simulink model "GPESTN1"  (Simulink 6.1)
settings: Solver=ode45  StartTime=0.0  StopTime=1000.0  MaxStep=0.02  MinStep=0.005  RelTol=1e-3
values from neighbouring files (symbols this model uses):
  A_gpe = 2    [data_GPE.m]    (also in data_GPI.m)
  A_stn = 5    [data_GPI.m]    (also in data_STN.m)
  B_gpe = .08    (= 0.08)    [data_GPE.m]    (also in data_GPI.m)
  B_stn = 1    [data_GPI.m]    (also in data_STN.m)
  c_gpe = 1    [data_GPE.m]
  c_stn = 1    [data_STN.m]
  cag0 = i_v_16(177:192)    [launch_sysGPESTN1.m]    (also in launch_sysGPESTN1_GPEDBS.m)
  cas0 = i_v_16(65:80)    [launch_sysGPESTN1.m]    (also in launch_sysGPESTN1_GPEDBS.m)
  egpegpe = -80    [data_synapses.m]
  egpestn = -100    [data_synapses.m]
  ek_gpe = -80.0    (= -80)    [data_GPE.m]
  ek_stn = -80.0    (= -80)    [data_STN.m]
  el_gpe = -55.0    (= -55)    [data_GPE.m]
  el_stn = -60.0    (= -60)    [data_STN.m]
  epsil_gpe = 1*10^-4    (= 0.0001)    [data_GPE.m]
  epsil_stn = 3.75*10^-5    (= 3.75e-05)    [data_STN.m]
  estngpe = 0    [data_synapses.m]
  gahp_gpe = 30.0    (= 30)    [data_GPE.m]
  gahp_stn = 9.0    (= 9)    [data_STN.m]
  gca_gpe = 0.1    [data_GPE.m]
  gca_stn = 0.5    [data_STN.m]
  ggpegpe = .3    (= 0.3)    [data_synapses.m]    (also in launch_sysGPESTN1.m; launch_sysGPESTN1_GPEDBS.m = 0)
  ggpestn = .90    (= 0.9)    [data_synapses.m]
  gk_gpe = 30.0    (= 30)    [data_GPE.m]
  gk_stn = 45.0    (= 45)    [data_STN.m]
  gl_gpe = .1    (= 0.1)    [data_GPE.m]
  gl_stn = 2.25    [data_STN.m]
  gna_gpe = 120    [data_GPE.m]
  gna_stn = 37.5    [data_STN.m]
  gstngpe = .3    (= 0.3)    [data_synapses.m]
  gt_gpe = .5    (= 0.5)    [data_GPE.m]
  gt_stn = 0.5    [data_STN.m]
  hg0 = i_v_16(129:144)    [launch_sysGPESTN1.m]    (also in launch_sysGPESTN1_GPEDBS.m)
  hs0 = i_v_16(17:32)    [launch_sysGPESTN1.m]    (also in launch_sysGPESTN1_GPEDBS.m)
  k1_gpe = 30.0    (= 30)    [data_GPE.m]
  k1_stn = 15.0    (= 15)    [data_STN.m]
  kca_gpe = 15    [data_GPE.m]
  kca_stn = 22.5    [data_STN.m]
  ng0 = i_v_16(145:160)    [launch_sysGPESTN1.m]    (also in launch_sysGPESTN1_GPEDBS.m)
  ns0 = i_v_16(33:48)    [launch_sysGPESTN1.m]    (also in launch_sysGPESTN1_GPEDBS.m)
  phih_gpe = 0.05    [data_GPE.m]
  phih_stn = 0.75    [data_STN.m]
  phin_gpe = 0.1    [data_GPE.m]
  phin_stn = 0.75    [data_STN.m]
  phir_gpe = 1    [data_GPE.m]
  phir_stn = 0.5    [data_STN.m]
  rg0 = i_v_16(161:176)    [launch_sysGPESTN1.m]    (also in launch_sysGPESTN1_GPEDBS.m)
  rs0 = i_v_16(49:64)    [launch_sysGPESTN1.m]    (also in launch_sysGPESTN1_GPEDBS.m)
  sg0 = i_v_16(193:208)    [launch_sysGPESTN1.m]    (also in launch_sysGPESTN1_GPEDBS.m)
  sigmaa_gpe = 2    [data_GPE.m]
  sigmaa_stn = 7.8    [data_STN.m]
  sigmab_stn = -0.07    [data_STN.m]
  sigmagh_gpe = 2.0    (= 2)    [data_GPE.m]
  sigmagh_stn = 8.0    (= 8)    [data_STN.m]
  sigmah_gpe = -12    [data_GPE.m]
  sigmah_stn = -3.1    [data_STN.m]
  sigmam_gpe = 10.0    (= 10)    [data_GPE.m]
  sigmam_stn = 15.0    (= 15)    [data_STN.m]
  sigman_gpe = 14.0    (= 14)    [data_GPE.m]
  sigman_stn = 8.0    (= 8)    [data_STN.m]
  sigmar_gpe = -2.0    (= -2)    [data_GPE.m]
  sigmar_stn = -2.0    (= -2)    [data_STN.m]
  sigmas_gpe = 2    [data_GPE.m]
  sigmas_stn = 8.0    (= 8)    [data_STN.m]
  sigmatauh_gpe = -12    [data_GPE.m]
  sigmatauh_stn = -3.0    (= -3)    [data_STN.m]
  sigmataun_gpe = -12.0    (= -12)    [data_GPE.m]
  sigmataun_stn = -26.0    (= -26)    [data_STN.m]
  sigmataur_stn = -2.2    [data_STN.m]
  ss0 = i_v_16(81:96)    [launch_sysGPESTN1.m]    (also in launch_sysGPESTN1_GPEDBS.m)
  syn_stngpe_gain = .2    (= 0.2)    [data_STN.m]
  tauh0_gpe = .05    (= 0.05)    [data_GPE.m]
  tauh0_stn = 1.0    (= 1)    [data_STN.m]
  tauh1_gpe = .27    (= 0.27)    [data_GPE.m]
  tauh1_stn = 500.0    (= 500)    [data_STN.m]
  taun0_gpe = .05    (= 0.05)    [data_GPE.m]
  taun0_stn = 1.0    (= 1)    [data_STN.m]
  taun1_gpe = .27    (= 0.27)    [data_GPE.m]
  taun1_stn = 100.0    (= 100)    [data_STN.m]
  taur0_stn = 7.1    [data_STN.m]
  taur1_stn = 17.5    [data_STN.m]
  taur_gpe = 30.0    (= 30)    [data_GPE.m]
  theta_gpe = 20    [data_GPE.m]    (also in data_GPI.m)
  theta_stn = 30    [data_GPI.m]    (also in data_STN.m)
  thetaa_gpe = -57.0    (= -57)    [data_GPE.m]
  thetaa_stn = -63.0    (= -63)    [data_STN.m]
  thetab_stn = 0.25    [data_STN.m]
  thetagh_gpe = -57.0    (= -57)    [data_GPE.m]
  thetagh_stn = -39.0    (= -39)    [data_STN.m]
  thetah_gpe = -58.0    (= -58)    [data_GPE.m]
  thetah_stn = -39.0    (= -39)    [data_STN.m]
  thetam_gpe = -37.0    (= -37)    [data_GPE.m]
  thetam_stn = -30.0    (= -30)    [data_STN.m]
  thetan_gpe = -50.0    (= -50)    [data_GPE.m]
  thetan_stn = -32.0    (= -32)    [data_STN.m]
  thetar_gpe = -70.0    (= -70)    [data_GPE.m]
  thetar_stn = -67.0    (= -67)    [data_STN.m]
  thetas_gpe = -35.0    (= -35)    [data_GPE.m]
  thetas_stn = -39.0    (= -39)    [data_STN.m]
  thetatauh_gpe = -40.0    (= -40)    [data_GPE.m]
  thetatauh_stn = -57.0    (= -57)    [data_STN.m]
  thetataun_gpe = -40.0    (= -40)    [data_GPE.m]
  thetataun_stn = -80.0    (= -80)    [data_STN.m]
  thetataur_stn = 68.0    (= 68)    [data_STN.m]
  vg0 = i_v_16(113:128)    [launch_sysGPESTN1.m]    (also in launch_sysGPESTN1_GPEDBS.m)
  vs0 = i_v_16(1:16)    [launch_sysGPESTN1.m]    (also in launch_sysGPESTN1_GPEDBS.m)
undefined symbols (not defined in the file or in its folder): cag01, cas01, hg01, hs01, ng01, ns01, rg01, rs01, sg01, ss01, vg01, vs01
(part 2 of 9)

== system GPESTN1/igpegpe4 ==
  In1 : Inport  Port=1  LatchInput=off
  In2 : Inport  Port=2  LatchInput=off
  In3 : Inport  Port=3  LatchInput=off
  Fcn : Fcn  Expr=ggpegpe*(u-egpegpe)
  Product : Product  SaturateOnIntegerOverflow=on  InputSameDT=on
  Sum : Sum  SaturateOnIntegerOverflow=on  InputSameDT=on
  Out1 : Outport
  wires:
  Sum/1 -> Product/1
  Fcn/1 -> Product/2
  In1/1 -> Sum/1
  In2/1 -> Sum/2
  Product/1 -> Out1/1
  In3/1 -> Fcn/1

== system GPESTN1/igpegpe5 ==
  In1 : Inport  Port=1  LatchInput=off
  In2 : Inport  Port=2  LatchInput=off
  In3 : Inport  Port=3  LatchInput=off
  Fcn : Fcn  Expr=ggpegpe*(u-egpegpe)
  Product : Product  SaturateOnIntegerOverflow=on  InputSameDT=on
  Sum : Sum  SaturateOnIntegerOverflow=on  InputSameDT=on
  Out1 : Outport
  wires:
  Sum/1 -> Product/1
  Fcn/1 -> Product/2
  In1/1 -> Sum/1
  In2/1 -> Sum/2
  Product/1 -> Out1/1
  In3/1 -> Fcn/1

== system GPESTN1/igpegpe6 ==
  In1 : Inport  Port=1  LatchInput=off
  In2 : Inport  Port=2  LatchInput=off
  In3 : Inport  Port=3  LatchInput=off
  Fcn : Fcn  Expr=ggpegpe*(u-egpegpe)
  Product : Product  SaturateOnIntegerOverflow=on  InputSameDT=on
  Sum : Sum  SaturateOnIntegerOverflow=on  InputSameDT=on
  Out1 : Outport
  wires:
  Sum/1 -> Product/1
  Fcn/1 -> Product/2
  In1/1 -> Sum/1
  In2/1 -> Sum/2
  Product/1 -> Out1/1
  In3/1 -> Fcn/1

== system GPESTN1/igpegpe7 ==
  In1 : Inport  Port=1  LatchInput=off
  In2 : Inport  Port=2  LatchInput=off
  In3 : Inport  Port=3  LatchInput=off
  Fcn : Fcn  Expr=ggpegpe*(u-egpegpe)
  Product : Product  SaturateOnIntegerOverflow=on  InputSameDT=on
  Sum : Sum  SaturateOnIntegerOverflow=on  InputSameDT=on
  Out1 : Outport
  wires:
  Sum/1 -> Product/1
  Fcn/1 -> Product/2
  In1/1 -> Sum/1
  In2/1 -> Sum/2
  Product/1 -> Out1/1
  In3/1 -> Fcn/1

== system GPESTN1/igpegpe8 ==
  In1 : Inport  Port=1  LatchInput=off
  In2 : Inport  Port=2  LatchInput=off
  In3 : Inport  Port=3  LatchInput=off
  Fcn : Fcn  Expr=ggpegpe*(u-egpegpe)
  Product : Product  SaturateOnIntegerOverflow=on  InputSameDT=on
  Sum : Sum  SaturateOnIntegerOverflow=on  InputSameDT=on
  Out1 : Outport
  wires:
  Sum/1 -> Product/1
  Fcn/1 -> Product/2
  In1/1 -> Sum/1
  In2/1 -> Sum/2
  Product/1 -> Out1/1
  In3/1 -> Fcn/1

== system GPESTN1/igpegpe9 ==
  In1 : Inport  Port=1  LatchInput=off
  In2 : Inport  Port=2  LatchInput=off
  In3 : Inport  Port=3  LatchInput=off
  Fcn : Fcn  Expr=ggpegpe*(u-egpegpe)
  Product : Product  SaturateOnIntegerOverflow=on  InputSameDT=on
  Sum : Sum  SaturateOnIntegerOverflow=on  InputSameDT=on
  Out1 : Outport
  wires:
  Sum/1 -> Product/1
  Fcn/1 -> Product/2
  In1/1 -> Sum/1
  In2/1 -> Sum/2
  Product/1 -> Out1/1
  In3/1 -> Fcn/1

== system GPESTN1/igpestn ==
  In1 : Inport  Port=1  LatchInput=off
  In2 : Inport  Port=2  LatchInput=off
  In3 : Inport  Port=3  LatchInput=off
  Fcn : Fcn  Expr=ggpestn*(u-egpestn)
  Product : Product  SaturateOnIntegerOverflow=on  InputSameDT=on
  Sum : Sum  SaturateOnIntegerOverflow=on  InputSameDT=on
  Out1 : Outport
  wires:
  Sum/1 -> Product/1
  Fcn/1 -> Product/2
  In1/1 -> Sum/1
  In2/1 -> Sum/2
  Product/1 -> Out1/1
  In3/1 -> Fcn/1

== system GPESTN1/igpestn1 ==
  In1 : Inport  Port=1  LatchInput=off
  In2 : Inport  Port=2  LatchInput=off
  In3 : Inport  Port=3  LatchInput=off
  Fcn : Fcn  Expr=ggpestn*(u-egpestn)
  Product : Product  SaturateOnIntegerOverflow=on  InputSameDT=on
  Sum : Sum  SaturateOnIntegerOverflow=on  InputSameDT=on
  Out1 : Outport
  wires:
  Sum/1 -> Product/1
  Fcn/1 -> Product/2
  In1/1 -> Sum/1
  In2/1 -> Sum/2
  Product/1 -> Out1/1
  In3/1 -> Fcn/1

== system GPESTN1/igpestn10 ==
  In1 : Inport  Port=1  LatchInput=off
  In2 : Inport  Port=2  LatchInput=off
  In3 : Inport  Port=3  LatchInput=off
  Fcn : Fcn  Expr=ggpestn*(u-egpestn)
  Product : Product  SaturateOnIntegerOverflow=on  InputSameDT=on
  Sum : Sum  SaturateOnIntegerOverflow=on  InputSameDT=on
  Out1 : Outport
  wires:
  Sum/1 -> Product/1
  Fcn/1 -> Product/2
  In1/1 -> Sum/1
  In2/1 -> Sum/2
  Product/1 -> Out1/1
  In3/1 -> Fcn/1

== system GPESTN1/igpestn11 ==
  In1 : Inport  Port=1  LatchInput=off
  In2 : Inport  Port=2  LatchInput=off
  In3 : Inport  Port=3  LatchInput=off
  Fcn : Fcn  Expr=ggpestn*(u-egpestn)
  Product : Product  SaturateOnIntegerOverflow=on  InputSameDT=on
  Sum : Sum  SaturateOnIntegerOverflow=on  InputSameDT=on
  Out1 : Outport
  wires:
  Sum/1 -> Product/1
  Fcn/1 -> Product/2
  In1/1 -> Sum/1
  In2/1 -> Sum/2
  Product/1 -> Out1/1
  In3/1 -> Fcn/1

== system GPESTN1/igpestn12 ==
  In1 : Inport  Port=1  LatchInput=off
  In2 : Inport  Port=2  LatchInput=off
  In3 : Inport  Port=3  LatchInput=off
  Fcn : Fcn  Expr=ggpestn*(u-egpestn)
  Product : Product  SaturateOnIntegerOverflow=on  InputSameDT=on
  Sum : Sum  SaturateOnIntegerOverflow=on  InputSameDT=on
  Out1 : Outport
  wires:
  Sum/1 -> Product/1
  Fcn/1 -> Product/2
  In1/1 -> Sum/1
  In2/1 -> Sum/2
  Product/1 -> Out1/1
  In3/1 -> Fcn/1

== system GPESTN1/igpestn13 ==
  In1 : Inport  Port=1  LatchInput=off
  In2 : Inport  Port=2  LatchInput=off
  In3 : Inport  Port=3  LatchInput=off
  Fcn : Fcn  Expr=ggpestn*(u-egpestn)
  Product : Product  SaturateOnIntegerOverflow=on  InputSameDT=on
  Sum : Sum  SaturateOnIntegerOverflow=on  InputSameDT=on
  Out1 : Outport
  wires:
  Sum/1 -> Product/1
  Fcn/1 -> Product/2
  In1/1 -> Sum/1
  In2/1 -> Sum/2
  Product/1 -> Out1/1
  In3/1 -> Fcn/1

== system GPESTN1/igpestn14 ==
  In1 : Inport  Port=1  LatchInput=off
  In2 : Inport  Port=2  LatchInput=off
  In3 : Inport  Port=3  LatchInput=off
  Fcn : Fcn  Expr=ggpestn*(u-egpestn)
  Product : Product  SaturateOnIntegerOverflow=on  InputSameDT=on
  Sum : Sum  SaturateOnIntegerOverflow=on  InputSameDT=on
  Out1 : Outport
  wires:
  Sum/1 -> Product/1
  Fcn/1 -> Product/2
  In1/1 -> Sum/1
  In2/1 -> Sum/2
  Product/1 -> Out1/1
  In3/1 -> Fcn/1

== system GPESTN1/igpestn15 ==
  In1 : Inport  Port=1  LatchInput=off
  In2 : Inport  Port=2  LatchInput=off
  In3 : Inport  Port=3  LatchInput=off
  Fcn : Fcn  Expr=ggpestn*(u-egpestn)
  Product : Product  SaturateOnIntegerOverflow=on  InputSameDT=on
  Sum : Sum  SaturateOnIntegerOverflow=on  InputSameDT=on
  Out1 : Outport
  wires:
  Sum/1 -> Product/1
  Fcn/1 -> Product/2
  In1/1 -> Sum/1
  In2/1 -> Sum/2
  Product/1 -> Out1/1
  In3/1 -> Fcn/1

== system GPESTN1/igpestn2 ==
  In1 : Inport  Port=1  LatchInput=off
  In2 : Inport  Port=2  LatchInput=off
  In3 : Inport  Port=3  LatchInput=off
  Fcn : Fcn  Expr=ggpestn*(u-egpestn)
  Product : Product  SaturateOnIntegerOverflow=on  InputSameDT=on
  Sum : Sum  SaturateOnIntegerOverflow=on  InputSameDT=on
  Out1 : Outport
  wires:
  Sum/1 -> Product/1
  Fcn/1 -> Product/2
  In1/1 -> Sum/1
  In2/1 -> Sum/2
  Product/1 -> Out1/1
  In3/1 -> Fcn/1

== system GPESTN1/igpestn3 ==
  In1 : Inport  Port=1  LatchInput=off
  In2 : Inport  Port=2  LatchInput=off
  In3 : Inport  Port=3  LatchInput=off
  Fcn : Fcn  Expr=ggpestn*(u-egpestn)
  Product : Product  SaturateOnIntegerOverflow=on  InputSameDT=on
  Sum : Sum  SaturateOnIntegerOverflow=on  InputSameDT=on
  Out1 : Outport
  wires:
  Sum/1 -> Product/1
  Fcn/1 -> Product/2
  In1/1 -> Sum/1
  In2/1 -> Sum/2
  Product/1 -> Out1/1
  In3/1 -> Fcn/1

== system GPESTN1/igpestn4 ==
  In1 : Inport  Port=1  LatchInput=off
  In2 : Inport  Port=2  LatchInput=off
  In3 : Inport  Port=3  LatchInput=off
  Fcn : Fcn  Expr=ggpestn*(u-egpestn)
  Product : Product  SaturateOnIntegerOverflow=on  InputSameDT=on
  Sum : Sum  SaturateOnIntegerOverflow=on  InputSameDT=on
  Out1 : Outport
  wires:
  Sum/1 -> Product/1
  Fcn/1 -> Product/2
  In1/1 -> Sum/1
  In2/1 -> Sum/2
  Product/1 -> Out1/1
  In3/1 -> Fcn/1

== system GPESTN1/igpestn5 ==
  In1 : Inport  Port=1  LatchInput=off
  In2 : Inport  Port=2  LatchInput=off
  In3 : Inport  Port=3  LatchInput=off
  Fcn : Fcn  Expr=ggpestn*(u-egpestn)
  Product : Product  SaturateOnIntegerOverflow=on  InputSameDT=on
  Sum : Sum  SaturateOnIntegerOverflow=on  InputSameDT=on
  Out1 : Outport
  wires:
  Sum/1 -> Product/1
  Fcn/1 -> Product/2
  In1/1 -> Sum/1
  In2/1 -> Sum/2
  Product/1 -> Out1/1
  In3/1 -> Fcn/1

== system GPESTN1/igpestn6 ==
  In1 : Inport  Port=1  LatchInput=off
  In2 : Inport  Port=2  LatchInput=off
  In3 : Inport  Port=3  LatchInput=off
  Fcn : Fcn  Expr=ggpestn*(u-egpestn)
  Product : Product  SaturateOnIntegerOverflow=on  InputSameDT=on
  Sum : Sum  SaturateOnIntegerOverflow=on  InputSameDT=on
  Out1 : Outport
  wires:
  Sum/1 -> Product/1
  Fcn/1 -> Product/2
  In1/1 -> Sum/1
  In2/1 -> Sum/2
  Product/1 -> Out1/1
  In3/1 -> Fcn/1

== system GPESTN1/igpestn7 ==
  In1 : Inport  Port=1  LatchInput=off
  In2 : Inport  Port=2  LatchInput=off
  In3 : Inport  Port=3  LatchInput=off
  Fcn : Fcn  Expr=ggpestn*(u-egpestn)
  Product : Product  SaturateOnIntegerOverflow=on  InputSameDT=on
  Sum : Sum  SaturateOnIntegerOverflow=on  InputSameDT=on
  Out1 : Outport
  wires:
  Sum/1 -> Product/1
  Fcn/1 -> Product/2
  In1/1 -> Sum/1
  In2/1 -> Sum/2
  Product/1 -> Out1/1
  In3/1 -> Fcn/1

== system GPESTN1/igpestn8 ==
  In1 : Inport  Port=1  LatchInput=off
  In2 : Inport  Port=2  LatchInput=off
  In3 : Inport  Port=3  LatchInput=off
  Fcn : Fcn  Expr=ggpestn*(u-egpestn)
  Product : Product  SaturateOnIntegerOverflow=on  InputSameDT=on
  Sum : Sum  SaturateOnIntegerOverflow=on  InputSameDT=on
  Out1 : Outport
  wires:
  Sum/1 -> Product/1
  Fcn/1 -> Product/2
  In1/1 -> Sum/1
  In2/1 -> Sum/2
  Product/1 -> Out1/1
  In3/1 -> Fcn/1

== system GPESTN1/igpestn9 ==
  In1 : Inport  Port=1  LatchInput=off
  In2 : Inport  Port=2  LatchInput=off
  In3 : Inport  Port=3  LatchInput=off
  Fcn : Fcn  Expr=ggpestn*(u-egpestn)
  Product : Product  SaturateOnIntegerOverflow=on  InputSameDT=on
  Sum : Sum  SaturateOnIntegerOverflow=on  InputSameDT=on
  Out1 : Outport
  wires:
  Sum/1 -> Product/1
  Fcn/1 -> Product/2
  In1/1 -> Sum/1
  In2/1 -> Sum/2
  Product/1 -> Out1/1
  In3/1 -> Fcn/1

== system GPESTN1/istngpe1 ==
  In1 : Inport  Port=1  LatchInput=off
  In2 : Inport  Port=2  LatchInput=off
  In3 : Inport  Port=3  LatchInput=off
  In4 : Inport  Port=4  LatchInput=off
  Fcn : Fcn  Expr=gstngpe*(u-estngpe)
  Gain : Gain  Gain=syn_stngpe_gain
  Product : Product  SaturateOnIntegerOverflow=on  InputSameDT=on
  Sum : Sum  Inputs=+++  SaturateOnIntegerOverflow=on
  Out1 : Outport
  wires:
  Product/1 -> Out1/1
  In1/1 -> Fcn/1
  Fcn/1 -> Product/1
  In2/1 -> Sum/1
  Sum/1 -> Product/2
  In4/1 -> Sum/3
  Gain/1 -> Sum/2
  In3/1 -> Gain/1

== system GPESTN1/istngpe10 ==
  In1 : Inport  Port=1  LatchInput=off
  In2 : Inport  Port=2  LatchInput=off
  In3 : Inport  Port=3  LatchInput=off
  In4 : Inport  Port=4  LatchInput=off
  Fcn : Fcn  Expr=gstngpe*(u-estngpe)
  Gain : Gain  Gain=syn_stngpe_gain
  Product : Product  SaturateOnIntegerOverflow=on  InputSameDT=on
  Sum : Sum  Inputs=+++  SaturateOnIntegerOverflow=on
  Out1 : Outport
  wires:
  Product/1 -> Out1/1
  In1/1 -> Fcn/1
  Fcn/1 -> Product/1
  In2/1 -> Sum/1
  Sum/1 -> Product/2
  In4/1 -> Sum/3
  Gain/1 -> Sum/2
  In3/1 -> Gain/1

== system GPESTN1/istngpe11 ==
  In1 : Inport  Port=1  LatchInput=off
  In2 : Inport  Port=2  LatchInput=off
  In3 : Inport  Port=3  LatchInput=off
  In4 : Inport  Port=4  LatchInput=off
  Fcn : Fcn  Expr=gstngpe*(u-estngpe)
  Gain : Gain  Gain=syn_stngpe_gain
  Product : Product  SaturateOnIntegerOverflow=on  InputSameDT=on
  Sum : Sum  Inputs=+++  SaturateOnIntegerOverflow=on
  Out1 : Outport
  wires:
  Product/1 -> Out1/1
  In1/1 -> Fcn/1
  Fcn/1 -> Product/1
  In2/1 -> Sum/1
  Sum/1 -> Product/2
  In4/1 -> Sum/3
  Gain/1 -> Sum/2
  In3/1 -> Gain/1

== system GPESTN1/istngpe12 ==
  In1 : Inport  Port=1  LatchInput=off
  In2 : Inport  Port=2  LatchInput=off
  In3 : Inport  Port=3  LatchInput=off
  In4 : Inport  Port=4  LatchInput=off
  Fcn : Fcn  Expr=gstngpe*(u-estngpe)
  Gain : Gain  Gain=syn_stngpe_gain
  Product : Product  SaturateOnIntegerOverflow=on  InputSameDT=on
  Sum : Sum  Inputs=+++  SaturateOnIntegerOverflow=on
  Out1 : Outport
  wires:
  Product/1 -> Out1/1
  In1/1 -> Fcn/1
  Fcn/1 -> Product/1
  In2/1 -> Sum/1
  Sum/1 -> Product/2
  In4/1 -> Sum/3
  Gain/1 -> Sum/2
  In3/1 -> Gain/1

== system GPESTN1/istngpe13 ==
  In1 : Inport  Port=1  LatchInput=off
  In2 : Inport  Port=2  LatchInput=off
  In3 : Inport  Port=3  LatchInput=off
  In4 : Inport  Port=4  LatchInput=off
  Fcn : Fcn  Expr=gstngpe*(u-estngpe)
  Gain : Gain  Gain=syn_stngpe_gain
  Product : Product  SaturateOnIntegerOverflow=on  InputSameDT=on
  Sum : Sum  Inputs=+++  SaturateOnIntegerOverflow=on
  Out1 : Outport
  wires:
  Product/1 -> Out1/1
  In1/1 -> Fcn/1
  Fcn/1 -> Product/1
  In2/1 -> Sum/1
  Sum/1 -> Product/2
  In4/1 -> Sum/3
  Gain/1 -> Sum/2
  In3/1 -> Gain/1

== system GPESTN1/istngpe14 ==
  In1 : Inport  Port=1  LatchInput=off
  In2 : Inport  Port=2  LatchInput=off
  In3 : Inport  Port=3  LatchInput=off
  In4 : Inport  Port=4  LatchInput=off
  Fcn : Fcn  Expr=gstngpe*(u-estngpe)
  Gain : Gain  Gain=syn_stngpe_gain
  Product : Product  SaturateOnIntegerOverflow=on  InputSameDT=on
  Sum : Sum  Inputs=+++  SaturateOnIntegerOverflow=on
  Out1 : Outport
  wires:
  Product/1 -> Out1/1
  In1/1 -> Fcn/1
  Fcn/1 -> Product/1
  In2/1 -> Sum/1
  Sum/1 -> Product/2
  In4/1 -> Sum/3
  Gain/1 -> Sum/2
  In3/1 -> Gain/1

== system GPESTN1/istngpe15 ==
  In1 : Inport  Port=1  LatchInput=off
  In2 : Inport  Port=2  LatchInput=off
  In3 : Inport  Port=3  LatchInput=off
  In4 : Inport  Port=4  LatchInput=off
  Fcn : Fcn  Expr=gstngpe*(u-estngpe)
  Gain : Gain  Gain=syn_stngpe_gain
  Product : Product  SaturateOnIntegerOverflow=on  InputSameDT=on
  Sum : Sum  Inputs=+++  SaturateOnIntegerOverflow=on
  Out1 : Outport
  wires:
  Product/1 -> Out1/1
  In1/1 -> Fcn/1
  Fcn/1 -> Product/1
  In2/1 -> Sum/1
  Sum/1 -> Product/2
  In4/1 -> Sum/3
  Gain/1 -> Sum/2
  In3/1 -> Gain/1

== system GPESTN1/istngpe16 ==
  In1 : Inport  Port=1  LatchInput=off
  In2 : Inport  Port=2  LatchInput=off
  In3 : Inport  Port=3  LatchInput=off
  In4 : Inport  Port=4  LatchInput=off
  Fcn : Fcn  Expr=gstngpe*(u-estngpe)
  Gain : Gain  Gain=syn_stngpe_gain
  Product : Product  SaturateOnIntegerOverflow=on  InputSameDT=on
  Sum : Sum  Inputs=+++  SaturateOnIntegerOverflow=on
  Out1 : Outport
  wires:
  Product/1 -> Out1/1
  In1/1 -> Fcn/1
  Fcn/1 -> Product/1
  In2/1 -> Sum/1
  Sum/1 -> Product/2
  In4/1 -> Sum/3
  Gain/1 -> Sum/2
  In3/1 -> Gain/1

== system GPESTN1/istngpe2 ==
  In1 : Inport  Port=1  LatchInput=off
  In2 : Inport  Port=2  LatchInput=off
  In3 : Inport  Port=3  LatchInput=off
  In4 : Inport  Port=4  LatchInput=off
  Fcn : Fcn  Expr=gstngpe*(u-estngpe)
  Gain : Gain  Gain=syn_stngpe_gain
  Product : Product  SaturateOnIntegerOverflow=on  InputSameDT=on
  Sum : Sum  Inputs=+++  SaturateOnIntegerOverflow=on
  Out1 : Outport
  wires:
  Product/1 -> Out1/1
  In1/1 -> Fcn/1
  Fcn/1 -> Product/1
  In2/1 -> Sum/1
  Sum/1 -> Product/2
  In4/1 -> Sum/3
  Gain/1 -> Sum/2
  In3/1 -> Gain/1

== system GPESTN1/istngpe3 ==
  In1 : Inport  Port=1  LatchInput=off
  In2 : Inport  Port=2  LatchInput=off
  In3 : Inport  Port=3  LatchInput=off
  In4 : Inport  Port=4  LatchInput=off
  Fcn : Fcn  Expr=gstngpe*(u-estngpe)
  Gain : Gain  Gain=syn_stngpe_gain
  Product : Product  SaturateOnIntegerOverflow=on  InputSameDT=on
  Sum : Sum  Inputs=+++  SaturateOnIntegerOverflow=on
  Out1 : Outport
  wires:
  Product/1 -> Out1/1
  In1/1 -> Fcn/1
  Fcn/1 -> Product/1
  In2/1 -> Sum/1
  Sum/1 -> Product/2
  In4/1 -> Sum/3
  Gain/1 -> Sum/2
  In3/1 -> Gain/1

== system GPESTN1/istngpe4 ==
  In1 : Inport  Port=1  LatchInput=off
  In2 : Inport  Port=2  LatchInput=off
  In3 : Inport  Port=3  LatchInput=off
  In4 : Inport  Port=4  LatchInput=off
  Fcn : Fcn  Expr=gstngpe*(u-estngpe)
  Gain : Gain  Gain=syn_stngpe_gain
  Product : Product  SaturateOnIntegerOverflow=on  InputSameDT=on
  Sum : Sum  Inputs=+++  SaturateOnIntegerOverflow=on
  Out1 : Outport
  wires:
  Product/1 -> Out1/1
  In1/1 -> Fcn/1
  Fcn/1 -> Product/1
  In2/1 -> Sum/1
  Sum/1 -> Product/2
  In4/1 -> Sum/3
  Gain/1 -> Sum/2
  In3/1 -> Gain/1

== system GPESTN1/istngpe5 ==
  In1 : Inport  Port=1  LatchInput=off
  In2 : Inport  Port=2  LatchInput=off
  In3 : Inport  Port=3  LatchInput=off
  In4 : Inport  Port=4  LatchInput=off
  Fcn : Fcn  Expr=gstngpe*(u-estngpe)
  Gain : Gain  Gain=syn_stngpe_gain
  Product : Product  SaturateOnIntegerOverflow=on  InputSameDT=on
  Sum : Sum  Inputs=+++  SaturateOnIntegerOverflow=on
  Out1 : Outport
  wires:
  Product/1 -> Out1/1
  In1/1 -> Fcn/1
  Fcn/1 -> Product/1
  In2/1 -> Sum/1
  Sum/1 -> Product/2
  In4/1 -> Sum/3
  Gain/1 -> Sum/2
  In3/1 -> Gain/1

== system GPESTN1/istngpe6 ==
  In1 : Inport  Port=1  LatchInput=off
  In2 : Inport  Port=2  LatchInput=off
  In3 : Inport  Port=3  LatchInput=off
  In4 : Inport  Port=4  LatchInput=off
  Fcn : Fcn  Expr=gstngpe*(u-estngpe)
  Gain : Gain  Gain=syn_stngpe_gain
  Product : Product  SaturateOnIntegerOverflow=on  InputSameDT=on
  Sum : Sum  Inputs=+++  SaturateOnIntegerOverflow=on
  Out1 : Outport
  wires:
  Product/1 -> Out1/1
  In1/1 -> Fcn/1
  Fcn/1 -> Product/1
  In2/1 -> Sum/1
  Sum/1 -> Product/2
  In4/1 -> Sum/3
  Gain/1 -> Sum/2
  In3/1 -> Gain/1

== system GPESTN1/istngpe7 ==
  In1 : Inport  Port=1  LatchInput=off
  In2 : Inport  Port=2  LatchInput=off
  In3 : Inport  Port=3  LatchInput=off
  In4 : Inport  Port=4  LatchInput=off
  Fcn : Fcn  Expr=gstngpe*(u-estngpe)
  Gain : Gain  Gain=syn_stngpe_gain
  Product : Product  SaturateOnIntegerOverflow=on  InputSameDT=on
  Sum : Sum  Inputs=+++  SaturateOnIntegerOverflow=on
  Out1 : Outport
  wires:
  Product/1 -> Out1/1
  In1/1 -> Fcn/1
  Fcn/1 -> Product/1
  In2/1 -> Sum/1
  Sum/1 -> Product/2
  In4/1 -> Sum/3
  Gain/1 -> Sum/2
  In3/1 -> Gain/1

== system GPESTN1/istngpe8 ==
  In1 : Inport  Port=1  LatchInput=off
  In2 : Inport  Port=2  LatchInput=off
  In3 : Inport  Port=3  LatchInput=off
  In4 : Inport  Port=4  LatchInput=off
  Fcn : Fcn  Expr=gstngpe*(u-estngpe)
  Gain : Gain  Gain=syn_stngpe_gain
  Product : Product  SaturateOnIntegerOverflow=on  InputSameDT=on
  Sum : Sum  Inputs=+++  SaturateOnIntegerOverflow=on
  Out1 : Outport
  wires:
  Product/1 -> Out1/1
  In1/1 -> Fcn/1
  Fcn/1 -> Product/1
  In2/1 -> Sum/1
  Sum/1 -> Product/2
  In4/1 -> Sum/3
  Gain/1 -> Sum/2
  In3/1 -> Gain/1

== system GPESTN1/istngpe9 ==
  In1 : Inport  Port=1  LatchInput=off
  In2 : Inport  Port=2  LatchInput=off
  In3 : Inport  Port=3  LatchInput=off
  In4 : Inport  Port=4  LatchInput=off
  Fcn : Fcn  Expr=gstngpe*(u-estngpe)
  Gain : Gain  Gain=syn_stngpe_gain
  Product : Product  SaturateOnIntegerOverflow=on  InputSameDT=on
  Sum : Sum  Inputs=+++  SaturateOnIntegerOverflow=on
  Out1 : Outport
  wires:
  Product/1 -> Out1/1
  In1/1 -> Fcn/1
  Fcn/1 -> Product/1
  In2/1 -> Sum/1
  Sum/1 -> Product/2
  In4/1 -> Sum/3
  Gain/1 -> Sum/2
  In3/1 -> Gain/1

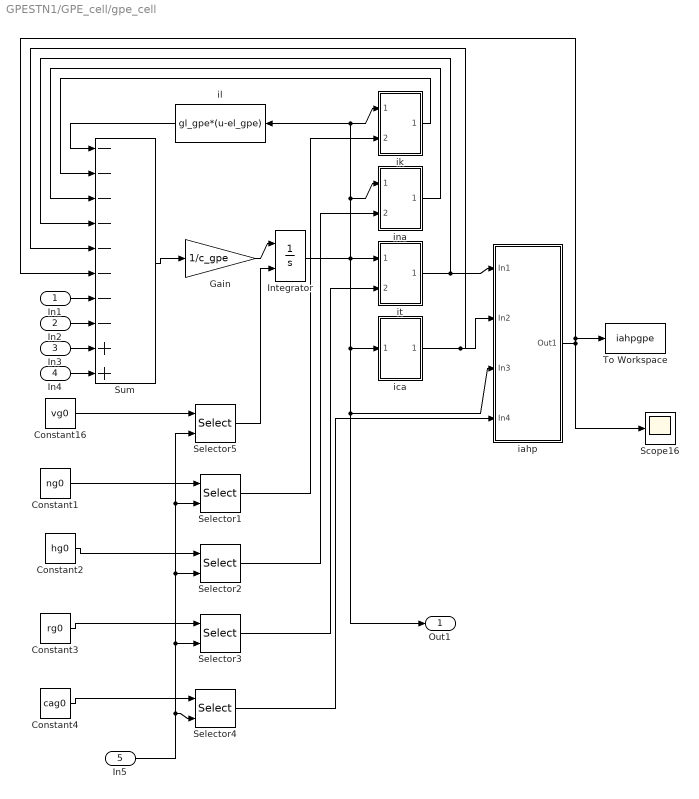
== system GPESTN1/GPE_cell/gpe_cell ==
  In1 : Inport  Port=1  LatchInput=off
  In2 : Inport  Port=2  LatchInput=off
  In3 : Inport  Port=3  LatchInput=off
  In4 : Inport  Port=4  LatchInput=off
  In5 : Inport  Port=5  LatchInput=off
  Constant1 : Constant  Value=ng0
  Constant16 : Constant  Value=vg0
  Constant2 : Constant  Value=hg0
  Constant3 : Constant  Value=rg0
  Constant4 : Constant  Value=cag0
  Gain : Gain  Gain=1/c_gpe  SaturateOnIntegerOverflow=on
  Integrator : Integrator  InitialConditionSource=external  InitialCondition=vg01  LimitOutput=on  UpperSaturationLimit=80
  Scope16 : Scope
      settings: YMin=-80  YMax=60  SaveName=ScopeData2
  Selector{1..5} (5 alike) : Selector  IndexMode=Zero-based  ElementSrc=External  Elements=[1 3]
  Sum : Sum  Description=--------  Inputs=--------++  SaturateOnIntegerOverflow=on  InputSameDT=on
  To Workspace : ToWorkspace  VariableName=iahpgpe  SampleTime=-1  SaveFormat=Structure
  iahp : Subsystem
  ica : Subsystem
  ik : Subsystem
  il : Fcn  Orientation=left  Expr=gl_gpe*(u-el_gpe)
  ina : Subsystem
  it : Subsystem
  Out1 : Outport
  wires:
  Gain/1 -> Integrator/1
  Sum/1 -> Gain/1
  Integrator/1 -> il/1, ik/1(In1), ina/1(In2), it/1(In2), ica/1(In1), iahp/3(In3), Out1/1
  il/1 -> Sum/1
  ik/1(Out1) -> Sum/2
  ina/1(Out1) -> Sum/3
  ica/1(Out1) -> Sum/5, iahp/2(In2)
  it/1(Out1) -> iahp/1(In1), Sum/4
  iahp/1(Out1) -> Sum/6, To Workspace/1, Scope16/1
  In1/1 -> Sum/7
  In2/1 -> Sum/8
  In3/1 -> Sum/9
  In4/1 -> Sum/10
  Constant4/1 -> Selector4/1
  Constant3/1 -> Selector3/1
  Constant2/1 -> Selector2/1
  Constant1/1 -> Selector1/1
  Constant16/1 -> Selector5/1
  In5/1 -> Selector5/2, Selector1/2, Selector2/2, Selector3/2, Selector4/2
  Selector5/1 -> Integrator/2
  Selector1/1 -> ik/2(In2)
  Selector2/1 -> ina/2(In1)
  Selector3/1 -> it/2(In1)
  Selector4/1 -> iahp/4(In4)

== system GPESTN1/GPE_cell/synap_gpe ==
  In1 : Inport  Port=1  LatchInput=off
  In2 : Inport  Port=2  LatchInput=off
  Fcn : Fcn  Expr=1/(1+exp(-(u-theta_gpe-thetagh_gpe)/sigmagh_gpe))
  Fcn2 : Fcn  Orientation=left  Expr=A_gpe*(1-u)
  Gain : Gain  Orientation=left  Gain=B_gpe  SaturateOnIntegerOverflow=on
  Integrator : Integrator  InitialConditionSource=external  InitialCondition=sg01
  Product : Product  SaturateOnIntegerOverflow=on  InputSameDT=on
  Sum : Sum  Inputs=|+-  SaturateOnIntegerOverflow=on  InputSameDT=on
  Out1 : Outport
  wires:
  Fcn/1 -> Product/1
  Fcn2/1 -> Product/2
  Product/1 -> Sum/1
  Sum/1 -> Integrator/1
  Integrator/1 -> Gain/1, Fcn2/1, Out1/1
  Gain/1 -> Sum/2
  In1/1 -> Fcn/1
  In2/1 -> Integrator/2

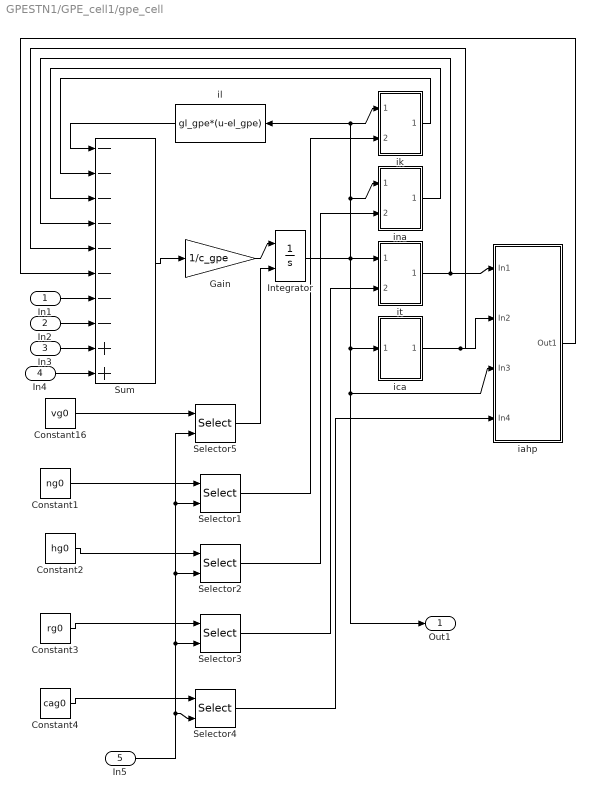
== system GPESTN1/GPE_cell1/gpe_cell ==
  In1 : Inport  Port=1  LatchInput=off
  In2 : Inport  Port=2  LatchInput=off
  In3 : Inport  Port=3  LatchInput=off
  In4 : Inport  Port=4  LatchInput=off
  In5 : Inport  Port=5  LatchInput=off
  Constant1 : Constant  Value=ng0
  Constant16 : Constant  Value=vg0
  Constant2 : Constant  Value=hg0
  Constant3 : Constant  Value=rg0
  Constant4 : Constant  Value=cag0
  Gain : Gain  Gain=1/c_gpe  SaturateOnIntegerOverflow=on
  Integrator : Integrator  InitialConditionSource=external  InitialCondition=vg01  LimitOutput=on  UpperSaturationLimit=80
  Selector{1..5} (5 alike) : Selector  IndexMode=Zero-based  ElementSrc=External  Elements=[1 3]
  Sum : Sum  Description=--------  Inputs=--------++  SaturateOnIntegerOverflow=on  InputSameDT=on
  iahp : Subsystem
  ica : Subsystem
  ik : Subsystem
  il : Fcn  Orientation=left  Expr=gl_gpe*(u-el_gpe)
  ina : Subsystem
  it : Subsystem
  Out1 : Outport
  wires:
  Gain/1 -> Integrator/1
  Sum/1 -> Gain/1
  Integrator/1 -> il/1, ik/1(In1), ina/1(In2), it/1(In2), ica/1(In1), iahp/3(In3), Out1/1
  il/1 -> Sum/1
  ik/1(Out1) -> Sum/2
  ina/1(Out1) -> Sum/3
  ica/1(Out1) -> Sum/5, iahp/2(In2)
  it/1(Out1) -> iahp/1(In1), Sum/4
  iahp/1(Out1) -> Sum/6
  In1/1 -> Sum/7
  In2/1 -> Sum/8
  In3/1 -> Sum/9
  In4/1 -> Sum/10
  Constant4/1 -> Selector4/1
  Constant3/1 -> Selector3/1
  Constant2/1 -> Selector2/1
  Constant1/1 -> Selector1/1
  Constant16/1 -> Selector5/1
  In5/1 -> Selector5/2, Selector1/2, Selector2/2, Selector3/2, Selector4/2
  Selector5/1 -> Integrator/2
  Selector1/1 -> ik/2(In2)
  Selector2/1 -> ina/2(In1)
  Selector3/1 -> it/2(In1)
  Selector4/1 -> iahp/4(In4)

== system GPESTN1/GPE_cell1/synap_gpe ==
  In1 : Inport  Port=1  LatchInput=off
  In2 : Inport  Port=2  LatchInput=off
  Fcn : Fcn  Expr=1/(1+exp(-(u-theta_gpe-thetagh_gpe)/sigmagh_gpe))
  Fcn2 : Fcn  Orientation=left  Expr=A_gpe*(1-u)
  Gain : Gain  Orientation=left  Gain=B_gpe  SaturateOnIntegerOverflow=on
  Integrator : Integrator  InitialConditionSource=external  InitialCondition=sg01
  Product : Product  SaturateOnIntegerOverflow=on  InputSameDT=on
  Sum : Sum  Inputs=|+-  SaturateOnIntegerOverflow=on  InputSameDT=on
  Out1 : Outport
  wires:
  Fcn/1 -> Product/1
  Fcn2/1 -> Product/2
  Product/1 -> Sum/1
  Sum/1 -> Integrator/1
  Integrator/1 -> Gain/1, Fcn2/1, Out1/1
  Gain/1 -> Sum/2
  In1/1 -> Fcn/1
  In2/1 -> Integrator/2

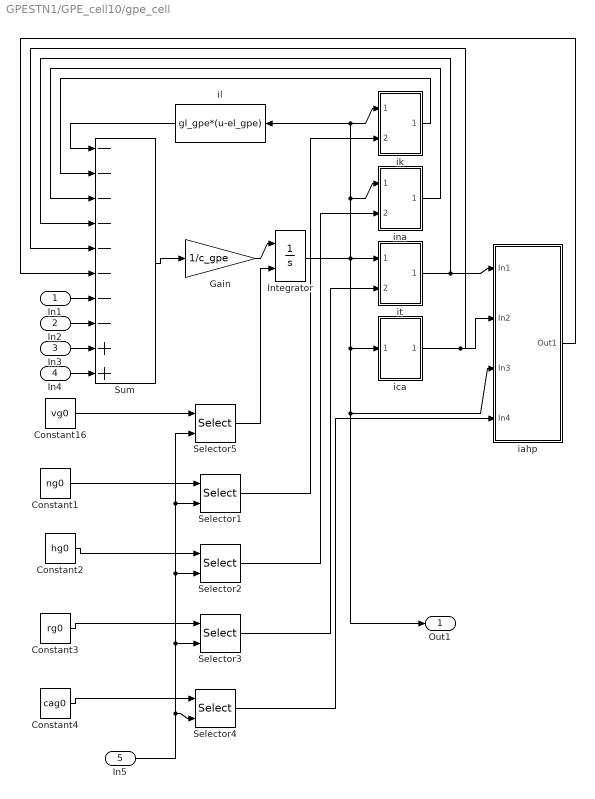
== system GPESTN1/GPE_cell10/gpe_cell ==
  In1 : Inport  Port=1  LatchInput=off
  In2 : Inport  Port=2  LatchInput=off
  In3 : Inport  Port=3  LatchInput=off
  In4 : Inport  Port=4  LatchInput=off
  In5 : Inport  Port=5  LatchInput=off
  Constant1 : Constant  Value=ng0
  Constant16 : Constant  Value=vg0
  Constant2 : Constant  Value=hg0
  Constant3 : Constant  Value=rg0
  Constant4 : Constant  Value=cag0
  Gain : Gain  Gain=1/c_gpe  SaturateOnIntegerOverflow=on
  Integrator : Integrator  InitialConditionSource=external  InitialCondition=vg01  LimitOutput=on  UpperSaturationLimit=80
  Selector{1..5} (5 alike) : Selector  IndexMode=Zero-based  ElementSrc=External  Elements=[1 3]
  Sum : Sum  Description=--------  Inputs=--------++  SaturateOnIntegerOverflow=on  InputSameDT=on
  iahp : Subsystem
  ica : Subsystem
  ik : Subsystem
  il : Fcn  Orientation=left  Expr=gl_gpe*(u-el_gpe)
  ina : Subsystem
  it : Subsystem
  Out1 : Outport
  wires:
  Gain/1 -> Integrator/1
  Sum/1 -> Gain/1
  Integrator/1 -> il/1, ik/1(In1), ina/1(In2), it/1(In2), ica/1(In1), iahp/3(In3), Out1/1
  il/1 -> Sum/1
  ik/1(Out1) -> Sum/2
  ina/1(Out1) -> Sum/3
  ica/1(Out1) -> Sum/5, iahp/2(In2)
  it/1(Out1) -> iahp/1(In1), Sum/4
  iahp/1(Out1) -> Sum/6
  In1/1 -> Sum/7
  In2/1 -> Sum/8
  In3/1 -> Sum/9
  In4/1 -> Sum/10
  Constant4/1 -> Selector4/1
  Constant3/1 -> Selector3/1
  Constant2/1 -> Selector2/1
  Constant1/1 -> Selector1/1
  Constant16/1 -> Selector5/1
  In5/1 -> Selector5/2, Selector1/2, Selector2/2, Selector3/2, Selector4/2
  Selector5/1 -> Integrator/2
  Selector1/1 -> ik/2(In2)
  Selector2/1 -> ina/2(In1)
  Selector3/1 -> it/2(In1)
  Selector4/1 -> iahp/4(In4)

== system GPESTN1/GPE_cell10/synap_gpe ==
  In1 : Inport  Port=1  LatchInput=off
  In2 : Inport  Port=2  LatchInput=off
  Fcn : Fcn  Expr=1/(1+exp(-(u-theta_gpe-thetagh_gpe)/sigmagh_gpe))
  Fcn2 : Fcn  Orientation=left  Expr=A_gpe*(1-u)
  Gain : Gain  Orientation=left  Gain=B_gpe  SaturateOnIntegerOverflow=on
  Integrator : Integrator  InitialConditionSource=external  InitialCondition=sg01
  Product : Product  SaturateOnIntegerOverflow=on  InputSameDT=on
  Sum : Sum  Inputs=|+-  SaturateOnIntegerOverflow=on  InputSameDT=on
  Out1 : Outport
  wires:
  Fcn/1 -> Product/1
  Fcn2/1 -> Product/2
  Product/1 -> Sum/1
  Sum/1 -> Integrator/1
  Integrator/1 -> Gain/1, Fcn2/1, Out1/1
  Gain/1 -> Sum/2
  In1/1 -> Fcn/1
  In2/1 -> Integrator/2

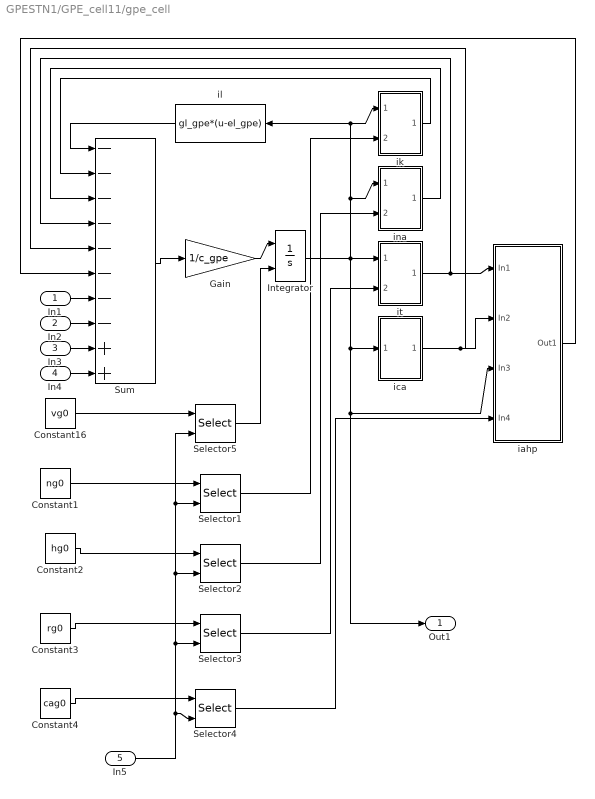
== system GPESTN1/GPE_cell11/gpe_cell ==
  In1 : Inport  Port=1  LatchInput=off
  In2 : Inport  Port=2  LatchInput=off
  In3 : Inport  Port=3  LatchInput=off
  In4 : Inport  Port=4  LatchInput=off
  In5 : Inport  Port=5  LatchInput=off
  Constant1 : Constant  Value=ng0
  Constant16 : Constant  Value=vg0
  Constant2 : Constant  Value=hg0
  Constant3 : Constant  Value=rg0
  Constant4 : Constant  Value=cag0
  Gain : Gain  Gain=1/c_gpe  SaturateOnIntegerOverflow=on
  Integrator : Integrator  InitialConditionSource=external  InitialCondition=vg01  LimitOutput=on  UpperSaturationLimit=80
  Selector{1..5} (5 alike) : Selector  IndexMode=Zero-based  ElementSrc=External  Elements=[1 3]
  Sum : Sum  Description=--------  Inputs=--------++  SaturateOnIntegerOverflow=on  InputSameDT=on
  iahp : Subsystem
  ica : Subsystem
  ik : Subsystem
  il : Fcn  Orientation=left  Expr=gl_gpe*(u-el_gpe)
  ina : Subsystem
  it : Subsystem
  Out1 : Outport
  wires:
  Gain/1 -> Integrator/1
  Sum/1 -> Gain/1
  Integrator/1 -> il/1, ik/1(In1), ina/1(In2), it/1(In2), ica/1(In1), iahp/3(In3), Out1/1
  il/1 -> Sum/1
  ik/1(Out1) -> Sum/2
  ina/1(Out1) -> Sum/3
  ica/1(Out1) -> Sum/5, iahp/2(In2)
  it/1(Out1) -> iahp/1(In1), Sum/4
  iahp/1(Out1) -> Sum/6
  In1/1 -> Sum/7
  In2/1 -> Sum/8
  In3/1 -> Sum/9
  In4/1 -> Sum/10
  Constant4/1 -> Selector4/1
  Constant3/1 -> Selector3/1
  Constant2/1 -> Selector2/1
  Constant1/1 -> Selector1/1
  Constant16/1 -> Selector5/1
  In5/1 -> Selector5/2, Selector1/2, Selector2/2, Selector3/2, Selector4/2
  Selector5/1 -> Integrator/2
  Selector1/1 -> ik/2(In2)
  Selector2/1 -> ina/2(In1)
  Selector3/1 -> it/2(In1)
  Selector4/1 -> iahp/4(In4)

== system GPESTN1/GPE_cell11/synap_gpe ==
  In1 : Inport  Port=1  LatchInput=off
  In2 : Inport  Port=2  LatchInput=off
  Fcn : Fcn  Expr=1/(1+exp(-(u-theta_gpe-thetagh_gpe)/sigmagh_gpe))
  Fcn2 : Fcn  Orientation=left  Expr=A_gpe*(1-u)
  Gain : Gain  Orientation=left  Gain=B_gpe  SaturateOnIntegerOverflow=on
  Integrator : Integrator  InitialConditionSource=external  InitialCondition=sg01
  Product : Product  SaturateOnIntegerOverflow=on  InputSameDT=on
  Sum : Sum  Inputs=|+-  SaturateOnIntegerOverflow=on  InputSameDT=on
  Out1 : Outport
  wires:
  Fcn/1 -> Product/1
  Fcn2/1 -> Product/2
  Product/1 -> Sum/1
  Sum/1 -> Integrator/1
  Integrator/1 -> Gain/1, Fcn2/1, Out1/1
  Gain/1 -> Sum/2
  In1/1 -> Fcn/1
  In2/1 -> Integrator/2

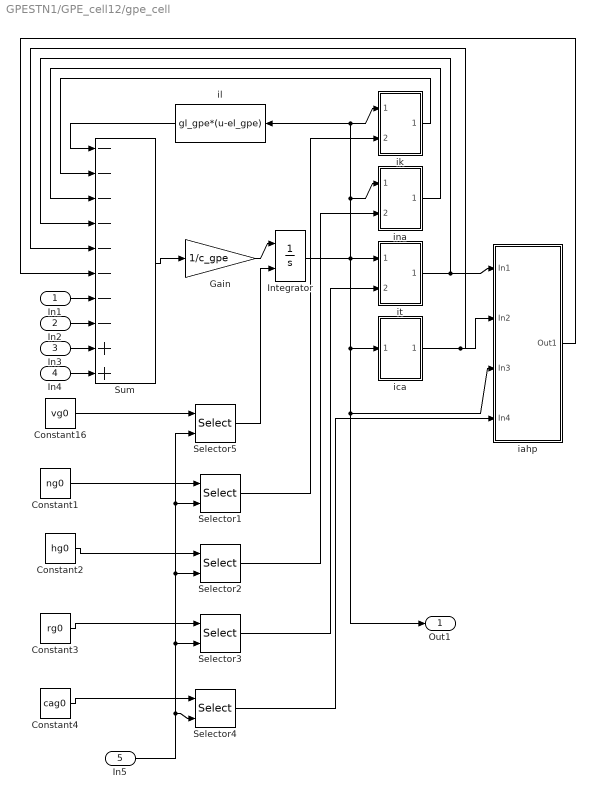
== system GPESTN1/GPE_cell12/gpe_cell ==
  In1 : Inport  Port=1  LatchInput=off
  In2 : Inport  Port=2  LatchInput=off
  In3 : Inport  Port=3  LatchInput=off
  In4 : Inport  Port=4  LatchInput=off
  In5 : Inport  Port=5  LatchInput=off
  Constant1 : Constant  Value=ng0
  Constant16 : Constant  Value=vg0
  Constant2 : Constant  Value=hg0
  Constant3 : Constant  Value=rg0
  Constant4 : Constant  Value=cag0
  Gain : Gain  Gain=1/c_gpe  SaturateOnIntegerOverflow=on
  Integrator : Integrator  InitialConditionSource=external  InitialCondition=vg01  LimitOutput=on  UpperSaturationLimit=80
  Selector{1..5} (5 alike) : Selector  IndexMode=Zero-based  ElementSrc=External  Elements=[1 3]
  Sum : Sum  Description=--------  Inputs=--------++  SaturateOnIntegerOverflow=on  InputSameDT=on
  iahp : Subsystem
  ica : Subsystem
  ik : Subsystem
  il : Fcn  Orientation=left  Expr=gl_gpe*(u-el_gpe)
  ina : Subsystem
  it : Subsystem
  Out1 : Outport
  wires:
  Gain/1 -> Integrator/1
  Sum/1 -> Gain/1
  Integrator/1 -> il/1, ik/1(In1), ina/1(In2), it/1(In2), ica/1(In1), iahp/3(In3), Out1/1
  il/1 -> Sum/1
  ik/1(Out1) -> Sum/2
  ina/1(Out1) -> Sum/3
  ica/1(Out1) -> Sum/5, iahp/2(In2)
  it/1(Out1) -> iahp/1(In1), Sum/4
  iahp/1(Out1) -> Sum/6
  In1/1 -> Sum/7
  In2/1 -> Sum/8
  In3/1 -> Sum/9
  In4/1 -> Sum/10
  Constant4/1 -> Selector4/1
  Constant3/1 -> Selector3/1
  Constant2/1 -> Selector2/1
  Constant1/1 -> Selector1/1
  Constant16/1 -> Selector5/1
  In5/1 -> Selector5/2, Selector1/2, Selector2/2, Selector3/2, Selector4/2
  Selector5/1 -> Integrator/2
  Selector1/1 -> ik/2(In2)
  Selector2/1 -> ina/2(In1)
  Selector3/1 -> it/2(In1)
  Selector4/1 -> iahp/4(In4)

== system GPESTN1/GPE_cell12/synap_gpe ==
  In1 : Inport  Port=1  LatchInput=off
  In2 : Inport  Port=2  LatchInput=off
  Fcn : Fcn  Expr=1/(1+exp(-(u-theta_gpe-thetagh_gpe)/sigmagh_gpe))
  Fcn2 : Fcn  Orientation=left  Expr=A_gpe*(1-u)
  Gain : Gain  Orientation=left  Gain=B_gpe  SaturateOnIntegerOverflow=on
  Integrator : Integrator  InitialConditionSource=external  InitialCondition=sg01
  Product : Product  SaturateOnIntegerOverflow=on  InputSameDT=on
  Sum : Sum  Inputs=|+-  SaturateOnIntegerOverflow=on  InputSameDT=on
  Out1 : Outport
  wires:
  Fcn/1 -> Product/1
  Fcn2/1 -> Product/2
  Product/1 -> Sum/1
  Sum/1 -> Integrator/1
  Integrator/1 -> Gain/1, Fcn2/1, Out1/1
  Gain/1 -> Sum/2
  In1/1 -> Fcn/1
  In2/1 -> Integrator/2

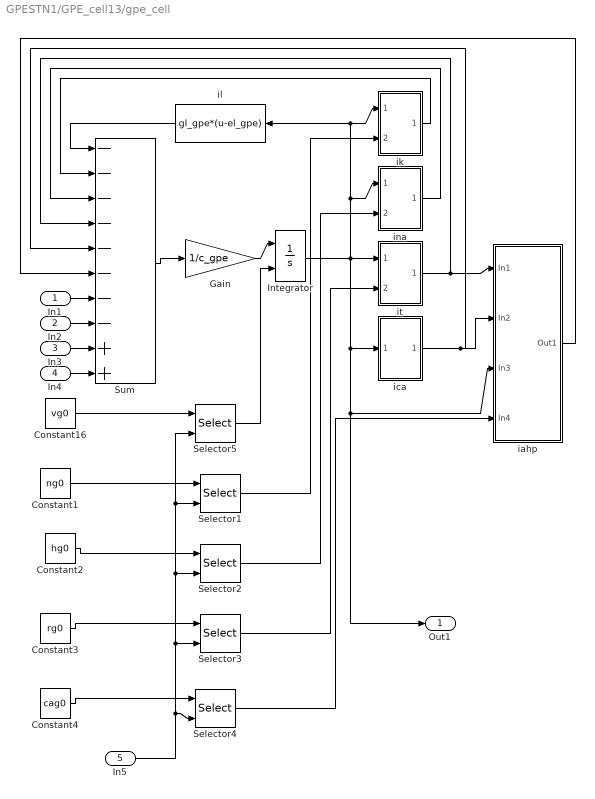
== system GPESTN1/GPE_cell13/gpe_cell ==
  In1 : Inport  Port=1  LatchInput=off
  In2 : Inport  Port=2  LatchInput=off
  In3 : Inport  Port=3  LatchInput=off
  In4 : Inport  Port=4  LatchInput=off
  In5 : Inport  Port=5  LatchInput=off
  Constant1 : Constant  Value=ng0
  Constant16 : Constant  Value=vg0
  Constant2 : Constant  Value=hg0
  Constant3 : Constant  Value=rg0
  Constant4 : Constant  Value=cag0
  Gain : Gain  Gain=1/c_gpe  SaturateOnIntegerOverflow=on
  Integrator : Integrator  InitialConditionSource=external  InitialCondition=vg01  LimitOutput=on  UpperSaturationLimit=80
  Selector{1..5} (5 alike) : Selector  IndexMode=Zero-based  ElementSrc=External  Elements=[1 3]
  Sum : Sum  Description=--------  Inputs=--------++  SaturateOnIntegerOverflow=on  InputSameDT=on
  iahp : Subsystem
  ica : Subsystem
  ik : Subsystem
  il : Fcn  Orientation=left  Expr=gl_gpe*(u-el_gpe)
  ina : Subsystem
  it : Subsystem
  Out1 : Outport
  wires:
  Gain/1 -> Integrator/1
  Sum/1 -> Gain/1
  Integrator/1 -> il/1, ik/1(In1), ina/1(In2), it/1(In2), ica/1(In1), iahp/3(In3), Out1/1
  il/1 -> Sum/1
  ik/1(Out1) -> Sum/2
  ina/1(Out1) -> Sum/3
  ica/1(Out1) -> Sum/5, iahp/2(In2)
  it/1(Out1) -> iahp/1(In1), Sum/4
  iahp/1(Out1) -> Sum/6
  In1/1 -> Sum/7
  In2/1 -> Sum/8
  In3/1 -> Sum/9
  In4/1 -> Sum/10
  Constant4/1 -> Selector4/1
  Constant3/1 -> Selector3/1
  Constant2/1 -> Selector2/1
  Constant1/1 -> Selector1/1
  Constant16/1 -> Selector5/1
  In5/1 -> Selector5/2, Selector1/2, Selector2/2, Selector3/2, Selector4/2
  Selector5/1 -> Integrator/2
  Selector1/1 -> ik/2(In2)
  Selector2/1 -> ina/2(In1)
  Selector3/1 -> it/2(In1)
  Selector4/1 -> iahp/4(In4)

== system GPESTN1/GPE_cell13/synap_gpe ==
  In1 : Inport  Port=1  LatchInput=off
  In2 : Inport  Port=2  LatchInput=off
  Fcn : Fcn  Expr=1/(1+exp(-(u-theta_gpe-thetagh_gpe)/sigmagh_gpe))
  Fcn2 : Fcn  Orientation=left  Expr=A_gpe*(1-u)
  Gain : Gain  Orientation=left  Gain=B_gpe  SaturateOnIntegerOverflow=on
  Integrator : Integrator  InitialConditionSource=external  InitialCondition=sg01
  Product : Product  SaturateOnIntegerOverflow=on  InputSameDT=on
  Sum : Sum  Inputs=|+-  SaturateOnIntegerOverflow=on  InputSameDT=on
  Out1 : Outport
  wires:
  Fcn/1 -> Product/1
  Fcn2/1 -> Product/2
  Product/1 -> Sum/1
  Sum/1 -> Integrator/1
  Integrator/1 -> Gain/1, Fcn2/1, Out1/1
  Gain/1 -> Sum/2
  In1/1 -> Fcn/1
  In2/1 -> Integrator/2

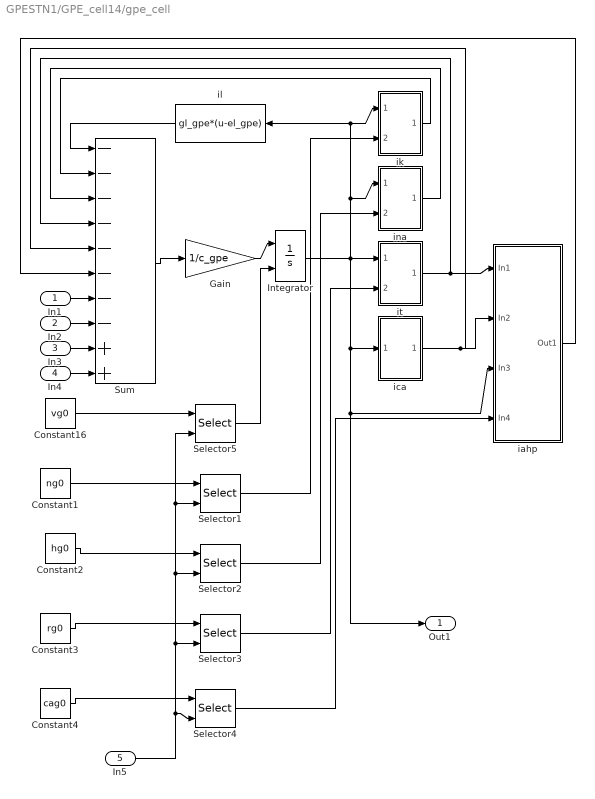
== system GPESTN1/GPE_cell14/gpe_cell ==
  In1 : Inport  Port=1  LatchInput=off
  In2 : Inport  Port=2  LatchInput=off
  In3 : Inport  Port=3  LatchInput=off
  In4 : Inport  Port=4  LatchInput=off
  In5 : Inport  Port=5  LatchInput=off
  Constant1 : Constant  Value=ng0
  Constant16 : Constant  Value=vg0
  Constant2 : Constant  Value=hg0
  Constant3 : Constant  Value=rg0
  Constant4 : Constant  Value=cag0
  Gain : Gain  Gain=1/c_gpe  SaturateOnIntegerOverflow=on
  Integrator : Integrator  InitialConditionSource=external  InitialCondition=vg01  LimitOutput=on  UpperSaturationLimit=80
  Selector{1..5} (5 alike) : Selector  IndexMode=Zero-based  ElementSrc=External  Elements=[1 3]
  Sum : Sum  Description=--------  Inputs=--------++  SaturateOnIntegerOverflow=on  InputSameDT=on
  iahp : Subsystem
  ica : Subsystem
  ik : Subsystem
  il : Fcn  Orientation=left  Expr=gl_gpe*(u-el_gpe)
  ina : Subsystem
  it : Subsystem
  Out1 : Outport
  wires:
  Gain/1 -> Integrator/1
  Sum/1 -> Gain/1
  Integrator/1 -> il/1, ik/1(In1), ina/1(In2), it/1(In2), ica/1(In1), iahp/3(In3), Out1/1
  il/1 -> Sum/1
  ik/1(Out1) -> Sum/2
  ina/1(Out1) -> Sum/3
  ica/1(Out1) -> Sum/5, iahp/2(In2)
  it/1(Out1) -> iahp/1(In1), Sum/4
  iahp/1(Out1) -> Sum/6
  In1/1 -> Sum/7
  In2/1 -> Sum/8
  In3/1 -> Sum/9
  In4/1 -> Sum/10
  Constant4/1 -> Selector4/1
  Constant3/1 -> Selector3/1
  Constant2/1 -> Selector2/1
  Constant1/1 -> Selector1/1
  Constant16/1 -> Selector5/1
  In5/1 -> Selector5/2, Selector1/2, Selector2/2, Selector3/2, Selector4/2
  Selector5/1 -> Integrator/2
  Selector1/1 -> ik/2(In2)
  Selector2/1 -> ina/2(In1)
  Selector3/1 -> it/2(In1)
  Selector4/1 -> iahp/4(In4)

== system GPESTN1/GPE_cell14/synap_gpe ==
  In1 : Inport  Port=1  LatchInput=off
  In2 : Inport  Port=2  LatchInput=off
  Fcn : Fcn  Expr=1/(1+exp(-(u-theta_gpe-thetagh_gpe)/sigmagh_gpe))
  Fcn2 : Fcn  Orientation=left  Expr=A_gpe*(1-u)
  Gain : Gain  Orientation=left  Gain=B_gpe  SaturateOnIntegerOverflow=on
  Integrator : Integrator  InitialConditionSource=external  InitialCondition=sg01
  Product : Product  SaturateOnIntegerOverflow=on  InputSameDT=on
  Sum : Sum  Inputs=|+-  SaturateOnIntegerOverflow=on  InputSameDT=on
  Out1 : Outport
  wires:
  Fcn/1 -> Product/1
  Fcn2/1 -> Product/2
  Product/1 -> Sum/1
  Sum/1 -> Integrator/1
  Integrator/1 -> Gain/1, Fcn2/1, Out1/1
  Gain/1 -> Sum/2
  In1/1 -> Fcn/1
  In2/1 -> Integrator/2

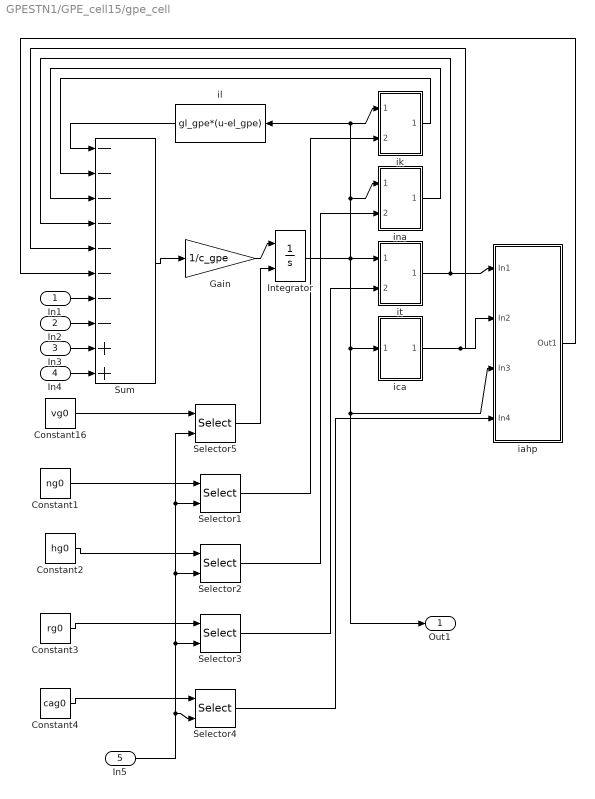
== system GPESTN1/GPE_cell15/gpe_cell ==
  In1 : Inport  Port=1  LatchInput=off
  In2 : Inport  Port=2  LatchInput=off
  In3 : Inport  Port=3  LatchInput=off
  In4 : Inport  Port=4  LatchInput=off
  In5 : Inport  Port=5  LatchInput=off
  Constant1 : Constant  Value=ng0
  Constant16 : Constant  Value=vg0
  Constant2 : Constant  Value=hg0
  Constant3 : Constant  Value=rg0
  Constant4 : Constant  Value=cag0
  Gain : Gain  Gain=1/c_gpe  SaturateOnIntegerOverflow=on
  Integrator : Integrator  InitialConditionSource=external  InitialCondition=vg01  LimitOutput=on  UpperSaturationLimit=80
  Selector{1..5} (5 alike) : Selector  IndexMode=Zero-based  ElementSrc=External  Elements=[1 3]
  Sum : Sum  Description=--------  Inputs=--------++  SaturateOnIntegerOverflow=on  InputSameDT=on
  iahp : Subsystem
  ica : Subsystem
  ik : Subsystem
  il : Fcn  Orientation=left  Expr=gl_gpe*(u-el_gpe)
  ina : Subsystem
  it : Subsystem
  Out1 : Outport
  wires:
  Gain/1 -> Integrator/1
  Sum/1 -> Gain/1
  Integrator/1 -> il/1, ik/1(In1), ina/1(In2), it/1(In2), ica/1(In1), iahp/3(In3), Out1/1
  il/1 -> Sum/1
  ik/1(Out1) -> Sum/2
  ina/1(Out1) -> Sum/3
  ica/1(Out1) -> Sum/5, iahp/2(In2)
  it/1(Out1) -> iahp/1(In1), Sum/4
  iahp/1(Out1) -> Sum/6
  In1/1 -> Sum/7
  In2/1 -> Sum/8
  In3/1 -> Sum/9
  In4/1 -> Sum/10
  Constant4/1 -> Selector4/1
  Constant3/1 -> Selector3/1
  Constant2/1 -> Selector2/1
  Constant1/1 -> Selector1/1
  Constant16/1 -> Selector5/1
  In5/1 -> Selector5/2, Selector1/2, Selector2/2, Selector3/2, Selector4/2
  Selector5/1 -> Integrator/2
  Selector1/1 -> ik/2(In2)
  Selector2/1 -> ina/2(In1)
  Selector3/1 -> it/2(In1)
  Selector4/1 -> iahp/4(In4)

== system GPESTN1/GPE_cell15/synap_gpe ==
  In1 : Inport  Port=1  LatchInput=off
  In2 : Inport  Port=2  LatchInput=off
  Fcn : Fcn  Expr=1/(1+exp(-(u-theta_gpe-thetagh_gpe)/sigmagh_gpe))
  Fcn2 : Fcn  Orientation=left  Expr=A_gpe*(1-u)
  Gain : Gain  Orientation=left  Gain=B_gpe  SaturateOnIntegerOverflow=on
  Integrator : Integrator  InitialConditionSource=external  InitialCondition=sg01
  Product : Product  SaturateOnIntegerOverflow=on  InputSameDT=on
  Sum : Sum  Inputs=|+-  SaturateOnIntegerOverflow=on  InputSameDT=on
  Out1 : Outport
  wires:
  Fcn/1 -> Product/1
  Fcn2/1 -> Product/2
  Product/1 -> Sum/1
  Sum/1 -> Integrator/1
  Integrator/1 -> Gain/1, Fcn2/1, Out1/1
  Gain/1 -> Sum/2
  In1/1 -> Fcn/1
  In2/1 -> Integrator/2

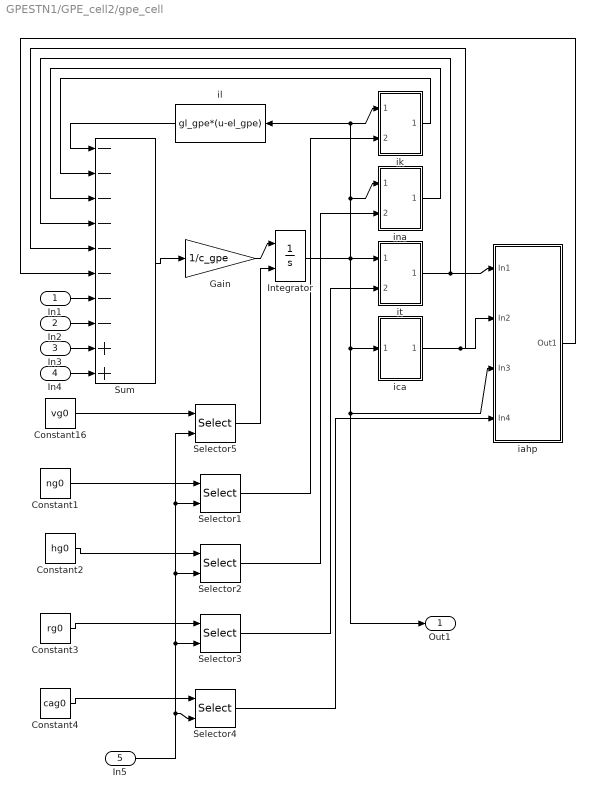
== system GPESTN1/GPE_cell2/gpe_cell ==
  In1 : Inport  Port=1  LatchInput=off
  In2 : Inport  Port=2  LatchInput=off
  In3 : Inport  Port=3  LatchInput=off
  In4 : Inport  Port=4  LatchInput=off
  In5 : Inport  Port=5  LatchInput=off
  Constant1 : Constant  Value=ng0
  Constant16 : Constant  Value=vg0
  Constant2 : Constant  Value=hg0
  Constant3 : Constant  Value=rg0
  Constant4 : Constant  Value=cag0
  Gain : Gain  Gain=1/c_gpe  SaturateOnIntegerOverflow=on
  Integrator : Integrator  InitialConditionSource=external  InitialCondition=vg01  LimitOutput=on  UpperSaturationLimit=80
  Selector{1..5} (5 alike) : Selector  IndexMode=Zero-based  ElementSrc=External  Elements=[1 3]
  Sum : Sum  Description=--------  Inputs=--------++  SaturateOnIntegerOverflow=on  InputSameDT=on
  iahp : Subsystem
  ica : Subsystem
  ik : Subsystem
  il : Fcn  Orientation=left  Expr=gl_gpe*(u-el_gpe)
  ina : Subsystem
  it : Subsystem
  Out1 : Outport
  wires:
  Gain/1 -> Integrator/1
  Sum/1 -> Gain/1
  Integrator/1 -> il/1, ik/1(In1), ina/1(In2), it/1(In2), ica/1(In1), iahp/3(In3), Out1/1
  il/1 -> Sum/1
  ik/1(Out1) -> Sum/2
  ina/1(Out1) -> Sum/3
  ica/1(Out1) -> Sum/5, iahp/2(In2)
  it/1(Out1) -> iahp/1(In1), Sum/4
  iahp/1(Out1) -> Sum/6
  In1/1 -> Sum/7
  In2/1 -> Sum/8
  In3/1 -> Sum/9
  In4/1 -> Sum/10
  Constant4/1 -> Selector4/1
  Constant3/1 -> Selector3/1
  Constant2/1 -> Selector2/1
  Constant1/1 -> Selector1/1
  Constant16/1 -> Selector5/1
  In5/1 -> Selector5/2, Selector1/2, Selector2/2, Selector3/2, Selector4/2
  Selector5/1 -> Integrator/2
  Selector1/1 -> ik/2(In2)
  Selector2/1 -> ina/2(In1)
  Selector3/1 -> it/2(In1)
  Selector4/1 -> iahp/4(In4)

== system GPESTN1/GPE_cell2/synap_gpe ==
  In1 : Inport  Port=1  LatchInput=off
  In2 : Inport  Port=2  LatchInput=off
  Fcn : Fcn  Expr=1/(1+exp(-(u-theta_gpe-thetagh_gpe)/sigmagh_gpe))
  Fcn2 : Fcn  Orientation=left  Expr=A_gpe*(1-u)
  Gain : Gain  Orientation=left  Gain=B_gpe  SaturateOnIntegerOverflow=on
  Integrator : Integrator  InitialConditionSource=external  InitialCondition=sg01
  Product : Product  SaturateOnIntegerOverflow=on  InputSameDT=on
  Sum : Sum  Inputs=|+-  SaturateOnIntegerOverflow=on  InputSameDT=on
  Out1 : Outport
  wires:
  Fcn/1 -> Product/1
  Fcn2/1 -> Product/2
  Product/1 -> Sum/1
  Sum/1 -> Integrator/1
  Integrator/1 -> Gain/1, Fcn2/1, Out1/1
  Gain/1 -> Sum/2
  In1/1 -> Fcn/1
  In2/1 -> Integrator/2

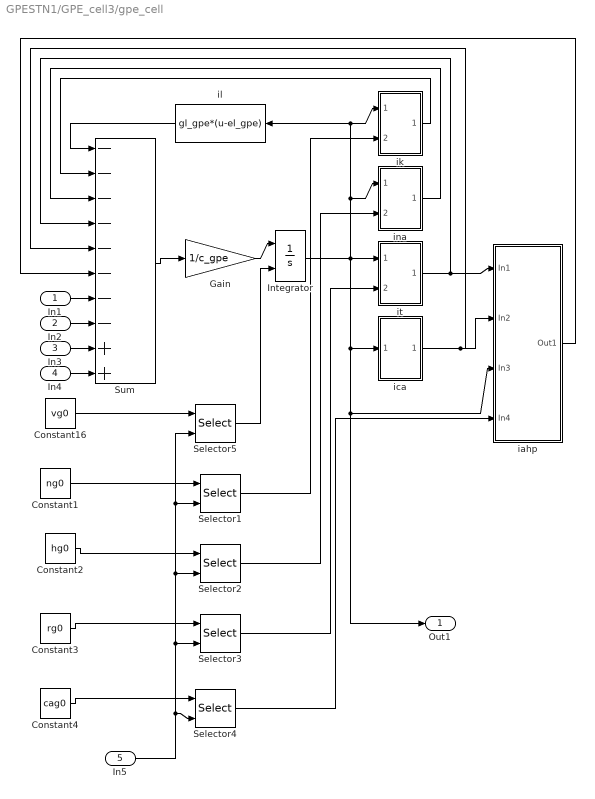
== system GPESTN1/GPE_cell3/gpe_cell ==
  In1 : Inport  Port=1  LatchInput=off
  In2 : Inport  Port=2  LatchInput=off
  In3 : Inport  Port=3  LatchInput=off
  In4 : Inport  Port=4  LatchInput=off
  In5 : Inport  Port=5  LatchInput=off
  Constant1 : Constant  Value=ng0
  Constant16 : Constant  Value=vg0
  Constant2 : Constant  Value=hg0
  Constant3 : Constant  Value=rg0
  Constant4 : Constant  Value=cag0
  Gain : Gain  Gain=1/c_gpe  SaturateOnIntegerOverflow=on
  Integrator : Integrator  InitialConditionSource=external  InitialCondition=vg01  LimitOutput=on  UpperSaturationLimit=80
  Selector{1..5} (5 alike) : Selector  IndexMode=Zero-based  ElementSrc=External  Elements=[1 3]
  Sum : Sum  Description=--------  Inputs=--------++  SaturateOnIntegerOverflow=on  InputSameDT=on
  iahp : Subsystem
  ica : Subsystem
  ik : Subsystem
  il : Fcn  Orientation=left  Expr=gl_gpe*(u-el_gpe)
  ina : Subsystem
  it : Subsystem
  Out1 : Outport
  wires:
  Gain/1 -> Integrator/1
  Sum/1 -> Gain/1
  Integrator/1 -> il/1, ik/1(In1), ina/1(In2), it/1(In2), ica/1(In1), iahp/3(In3), Out1/1
  il/1 -> Sum/1
  ik/1(Out1) -> Sum/2
  ina/1(Out1) -> Sum/3
  ica/1(Out1) -> Sum/5, iahp/2(In2)
  it/1(Out1) -> iahp/1(In1), Sum/4
  iahp/1(Out1) -> Sum/6
  In1/1 -> Sum/7
  In2/1 -> Sum/8
  In3/1 -> Sum/9
  In4/1 -> Sum/10
  Constant4/1 -> Selector4/1
  Constant3/1 -> Selector3/1
  Constant2/1 -> Selector2/1
  Constant1/1 -> Selector1/1
  Constant16/1 -> Selector5/1
  In5/1 -> Selector5/2, Selector1/2, Selector2/2, Selector3/2, Selector4/2
  Selector5/1 -> Integrator/2
  Selector1/1 -> ik/2(In2)
  Selector2/1 -> ina/2(In1)
  Selector3/1 -> it/2(In1)
  Selector4/1 -> iahp/4(In4)

== system GPESTN1/GPE_cell3/synap_gpe ==
  In1 : Inport  Port=1  LatchInput=off
  In2 : Inport  Port=2  LatchInput=off
  Fcn : Fcn  Expr=1/(1+exp(-(u-theta_gpe-thetagh_gpe)/sigmagh_gpe))
  Fcn2 : Fcn  Orientation=left  Expr=A_gpe*(1-u)
  Gain : Gain  Orientation=left  Gain=B_gpe  SaturateOnIntegerOverflow=on
  Integrator : Integrator  InitialConditionSource=external  InitialCondition=sg01
  Product : Product  SaturateOnIntegerOverflow=on  InputSameDT=on
  Sum : Sum  Inputs=|+-  SaturateOnIntegerOverflow=on  InputSameDT=on
  Out1 : Outport
  wires:
  Fcn/1 -> Product/1
  Fcn2/1 -> Product/2
  Product/1 -> Sum/1
  Sum/1 -> Integrator/1
  Integrator/1 -> Gain/1, Fcn2/1, Out1/1
  Gain/1 -> Sum/2
  In1/1 -> Fcn/1
  In2/1 -> Integrator/2
